simulink model "Increamental_Decreamental_counter"  (R2021a)
settings: Solver=VariableStepAuto  StartTime=0.0  StopTime=100  RelTol=1e-3
libraries: simulink x2
settings Model: Creator=Nour  LastModifiedBy=Nour

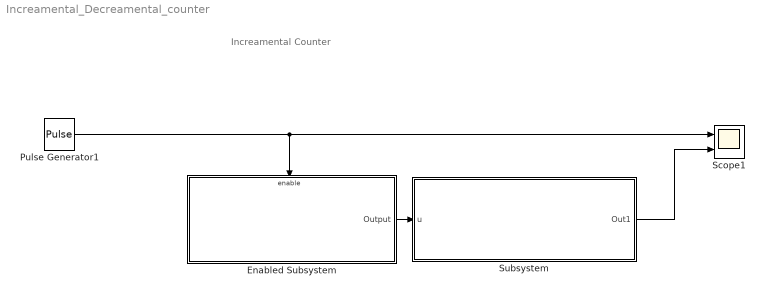
== system Increamental_Decreamental_counter ==
  note: Increamental Counter
  Enabled Subsystem : Subsystem  TreatAsAtomicUnit=on
  Pulse Generator1 : DiscretePulseGenerator  PulseType=Time based  Period=100  PulseWidth=50
  Scope1 : Scope  NumInputPorts=2
  Subsystem : Subsystem
  wires:
  Pulse Generator1/1 -> Scope1/1, Enabled Subsystem/Enable
  Enabled Subsystem/1(Output) -> Subsystem/1(u)
  Subsystem/1(Out1) -> Scope1/2

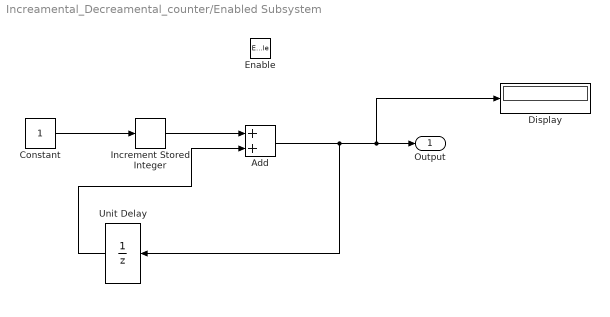
== system Increamental_Decreamental_counter/Enabled Subsystem ==
  Enable : EnablePort  StatesWhenEnabling=reset
  Add : Sum
  Constant : Constant
  Display : Display
  Increment Stored Integer : simulink/Additional Math & Discrete/Additional Math: Increment - Decrement/Increment Stored Integer
  Unit Delay : UnitDelay  SampleTime=-1  HasFrameUpgradeWarning=on
  Output : Outport
  wires:
  Unit Delay/1 -> Add/2
  Add/1 -> Unit Delay/1, Display/1, Output/1
  Constant/1 -> Increment Stored Integer/1
  Increment Stored Integer/1 -> Add/1

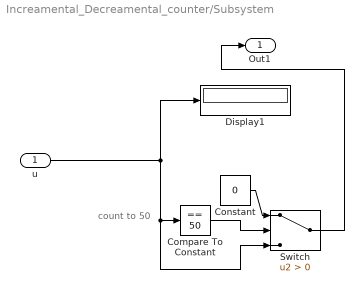
== system Increamental_Decreamental_counter/Subsystem ==
  note: count to 50
  u : Inport
  Compare To Constant : simulink/Logic and Bit Operations/Compare To Constant  relop===  const=50  OutDataTypeStr=boolean
  Constant : Constant  Value=0
  Display1 : Display
  Switch : Switch  Criteria=u2 > Threshold
  Out1 : Outport
  wires:
  u/1 -> Display1/1, Switch/3, Compare To Constant/1
  Constant/1 -> Switch/1
  Compare To Constant/1 -> Switch/2
  Switch/1 -> Out1/1
